simulink model "idmdlsim"  (Simulink 5.0)
settings: Solver=ode45  StartTime=0.0  StopTime=10  RelTol=1e-3
values from neighbouring files (symbols this model uses):
  A = s(1:2,1:2)    [motor.m]
  B = s(1:2,3)    [motor.m]
  C = eye(2)    [motor.m]
  D = D .* abs(ec{kexp}*ones(1,size(D,2)))    [arx.m]    (also in motor.m = [0;0])
  Ts = pvget(m0,'Ts')    [arx.m]    (also in idfilt.m = {1}; n4sid_f.m = {Ts}; predict.m = [])
  X0 = [0;0]    [motor.m]    (also in predict.m = X0*ones(1,Ne))
undefined symbols (not defined in the file or in its folder): idpoly
libraries: simulink x1
settings Model: Creator=jglass  LastModifiedBy=ljung  SignalLoggingName=logsOut  BlockReductionOpt=off  BooleanDataType=off  ZeroCrossControl=UseLocalSettings  RTWOptions="-aEnforceIntegerDowncast=1 -aFoldNonRolledExpr=1 -aInlineInvariantSignals=1 -aInlineParameters=0 -aLocalBlockOutputs=1 -aRollThreshold=5 -aRTWVerbose=1 -aGenerateReport=0 -aForceParamTrailComments=0 -aGenerateComments=1 -aIgnoreCustomStorageClasses=1 -aIncHierarchyInIds=0 -aMaxRTWIdLen=31 -aShowEliminatedStatements=0 -aReadOnly=0 -aTargetFcnLib=\"iso_c_tmw.mat\" -aIncDataTypeInIds=0 -aPrefixModelToSubsysFcnNames=1 -aInlinedPrmAccess=\"Literals\" -aGenerateFullHeader=1 -aIsPILTarget=0 -aLogVarNameModifier=\"rt_\" -aExtMode=0 -aExtModeStaticAlloc=0 -aExtModeTesting=0 -aExtModeStaticAllocSize=1000000 -aExtModeTransport=0"

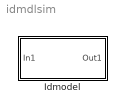
== system idmdlsim ==
  "Idmodel " : Subsystem  mask(Idmodel Block){sys=idpoly(1,1), IC=[], noi=on, seed=}
      mask prompts: sys "idmodel variable"; IC "Initial state (state space only: 'z', 'm', or vector )"; noi "Add noise"; seed "Noise seed(s)"
      mask help:
      | Enter any Idmodel object (Idpoly, Idss, Idarx, Idgrey or Idproc).
      | For simulations  with noise, Seed(s) may be left empty for random restarts. Enter a
      |  many seeds as there are outputs for specific realizations.
      mask init:
      | [A,B,C,D,Ts,X0,sysname]=idmdlmask('Initialize',gcb,sys,IC,noi,seed);
      mask Help:
      | The IDMODEL  block 	accepts any IDMODEL defined in the System Identification Toolbox: IDPOLY, IDSS,
      | IDGREY, IDARX and IDPROC. <p><P>
      | 
      | In the editiable text box enter the name of any IDMODEL in workspace.<p><p>
      | 
      |  For IDMODELS in state-space (IDSS and IDGREY) the initial state vector may be
      | specified. Use 'z' (within quotes) or 0 for zero initial conditions, use 'm' for the
      | Model's own initial state (I.e. MOD.X0) or specify the initial state  as a vector.<p><p>
      | 
      | To add noise to the simulation, check the corresponding box. Noise will be
      | added in accordance with the models noise specifications, i.e. MOD.NoiseVariance and
      | the matrices or polynomials that determine the color of the additive noise. <p><p>
      | 
      | For continuous time models the variance of the momentary noise term is infinite
      | in theory. You will see an appropriately bandlimited version, taking into account
      | the natural time constants of the system. You may think of the resulting simulated output
      | being filtered with a low-pass filter with a pass-band that does not distort the dynamics
      | from the input.<p><p>
      | 
      | IDMODELS with time-delays (MOD.InputDelay nonzero) are properly treated. Discrete time
      | models are convereted into models which take care of the delay explicitly, (thereby
      | extending also X0). For continuous time models a transport delay block is used.
      mask CallbackString: idmdlmask('MaskLTICallback',gcb)||idmdlmask('MaskLTICallback',gcb)|
      mask Display: disp(sysname)

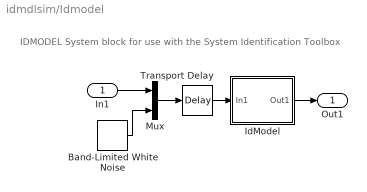
== system idmdlsim/Idmodel  ==
  note: IDMODEL System block
      | for use with the
      | System Identification Toolbox
  In1 : Inport
  Band-Limited White Noise : simulink/Sources/Band-Limited White Noise  Cov=1  Ts=1  seed=[-1364]
  IdModel : Subsystem
  Mux : Mux  Inputs=2
  Transport Delay : TransportDelay  DelayTime="[0  0]"
  Out1 : Outport
  wires:
  Band-Limited White Noise/1 -> Mux/2
  In1/1 -> Mux/1
  IdModel/1(Out1) -> Out1/1
  Transport Delay/1 -> IdModel/1(In1)
  Mux/1 -> Transport Delay/1

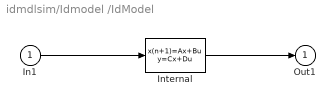
== system idmdlsim/Idmodel /IdModel ==
  In1 : Inport
  Internal : DiscreteStateSpace  A=A  B=B  C=C  D=D  X0=X0  SampleTime=Ts
  Out1 : Outport  InitialOutput=0
  wires:
  In1/1 -> Internal/1
  Internal/1 -> Out1/1
